simulink model "StepTesting"  (R2020a)
settings: Solver=FixedStepDiscrete  StartTime=0.0  StopTime=10.0  FixedStep=.001  RelTol=1e-3  EnableMultiTasking=on
settings Model: Creator=parham  LastModifiedBy=jhlim
settings DataIOCC: LimitDataPoints=on  SaveFormat=Array  SignalLoggingSaveFormat=ModelDataLogs  ReturnWorkspaceOutputs=off
settings OptimizationCC: ExpressionDepthLimit=2147483647  LifeSpan=inf
settings DebuggingCC: UnderspecifiedInitializationDetection=Classic  MergeDetectMultiDrivingBlocksExec=none  SolverPrmCheckMsg=warning  FcnCallInpInsideContextMsg=warning  StateNameClashWarn=warning  SFUnexpectedBacktrackingDiag=warning  SFNoUnconditionalDefaultTransitionDiag=warning  SFExecutionAtInitializationDiag=none  ArithmeticOperatorsInVariantConditions=warning
settings HardwareCC: ProdBitPerPointer=32  ProdBitPerSizeT=32  ProdBitPerPtrDiffT=32  ProdLargestAtomicFloat=None  ProdIntDivRoundTo=Undefined  ProdEndianess=Unspecified  ProdWordSize=32  ProdHWDeviceType=32-bit Generic
settings ModelReferenceCC: PropagateSignalLabelsOutOfModel=off
settings SFSimCC: SimUseLocalCustomCode=off  CustomCodeUndefinedFunction=UseInterfaceOnly
settings RTWCC: RTWUseLocalCustomCode=off
settings CodeAppCC: StateflowObjectComments=on
settings GRTTargetCC: TargetLangStandard=C89/C90 (ANSI)  CombineOutputUpdateFcns=off  GRTInterface=on
settings ConfigComp: CovMetricSettings=dw  CovHtmlReporting=on  CovSaveCumulativeToWorkspaceVar=on  CovSaveSingleToWorkspaceVar=on  CovExternalEMLEnable=off

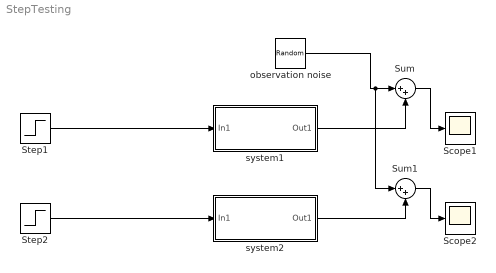
== system StepTesting ==
  Scope1 : Scope
  Scope2 : Scope
  Step1 : Step  Time=0  Before=1  SampleTime=.1
  Step2 : Step  Time=0  SampleTime=.1
  Sum : Sum  Inputs=|++
  Sum1 : Sum  Inputs=|++
  observation noise : RandomNumber  Variance=5  SampleTime=.1
  system1 : Subsystem
  system2 : Subsystem
  wires:
  system1/1(Out1) -> Sum/2
  observation noise/1 -> Sum/1, Sum1/1
  Sum/1 -> Scope1/1
  system2/1(Out1) -> Sum1/2
  Sum1/1 -> Scope2/1
  Step1/1 -> system1/1(In1)
  Step2/1 -> system2/1(In1)

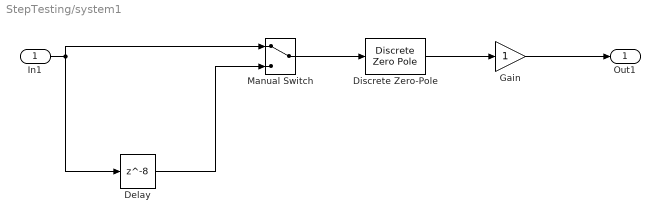
== system StepTesting/system1 ==
  In1 : Inport  SampleTime=.1
  Delay : Delay  DelayLength=8  SampleTime=.1
  Discrete Zero-Pole : DiscreteZeroPole  Zeros=[]  Poles=[0.9]  Gain=1  SampleTime=.1
  Gain : Gain  SampleTime=.1
  Manual Switch : ManualSwitch
  Out1 : Outport  SampleTime=.1
  wires:
  Discrete Zero-Pole/1 -> Gain/1
  Gain/1 -> Out1/1
  In1/1 -> Delay/1, Manual Switch/1
  Delay/1 -> Manual Switch/2
  Manual Switch/1 -> Discrete Zero-Pole/1

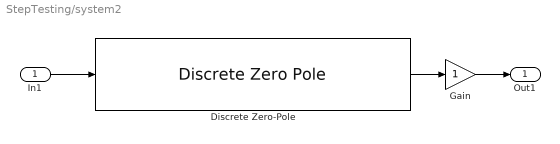
== system StepTesting/system2 ==
  In1 : Inport  SampleTime=.1
  Discrete Zero-Pole : DiscreteZeroPole  Zeros=[0.7261 ]  Poles=[0.7665+0.2705i 0.7665 - 0.2705i ]  Gain=0.4673  SampleTime=.1
  Gain : Gain  SampleTime=.1
  Out1 : Outport  SampleTime=.1
  wires:
  In1/1 -> Discrete Zero-Pole/1
  Discrete Zero-Pole/1 -> Gain/1
  Gain/1 -> Out1/1
